simulink model "hip_controller_2026_01_07"  (R2024b)
settings: Solver=FixedStepAuto  StartTime=0.0  StopTime=simDuration  FixedStep=0.01  RelTol=1e-3  EnableMultiTasking=on
InitFcn:
  | breakp=[-1, -0.8, -0.6, -0.4, -0.2, -0.1, 0, 0.1, 0.2, 0.4, 0.6, 0.8, 1];
  | splinenew =[-1, -0.8, -0.6, -0.4, -0.2, -0.1, 0, 0, 0.005, 0.01, 0.015,0.02,0.025];
undefined symbols (not defined in the file or in its folder): Discrete, K, qbreak, Time
libraries: simulink x53, arduinolib x11, dspswit3 x9, ctrlSharedLib x4, dspfdesign x2, slpidlib x2
(part 3 of 4)

== system hip_controller_2026_01_07/Subsystem3/Left Motor Velocity/Motor Actual Position Receive/CHINESE CORRECTION ==
  position : Inport
  Enable : EnablePort  StatesWhenEnabling=reset
  Abs : Abs  SaturateOnIntegerOverflow=off
  Constant2 : Constant
  Constant3 : Constant  Value=0
  Memory : Memory
  Subsystem : Subsystem
  Sum : Sum  Inputs=|+-
  Sum1 : Sum  Inputs=+-
  Switch1 : Switch  Criteria=u2 > Threshold  Threshold=20  SaturateOnIntegerOverflow=off  InputSameDT=off
  Out1 : Outport
  wires:
  Constant2/1 -> Switch1/1
  position/1 -> Sum1/1, Sum/1, Memory/1
  Sum/1 -> Abs/1, Subsystem/1(In1)
  Sum1/1 -> Out1/1
  Abs/1 -> Switch1/2
  Constant3/1 -> Switch1/3
  Switch1/1 -> Subsystem/Enable
  Memory/1 -> Sum/2
  Subsystem/1(Out1) -> Sum1/2

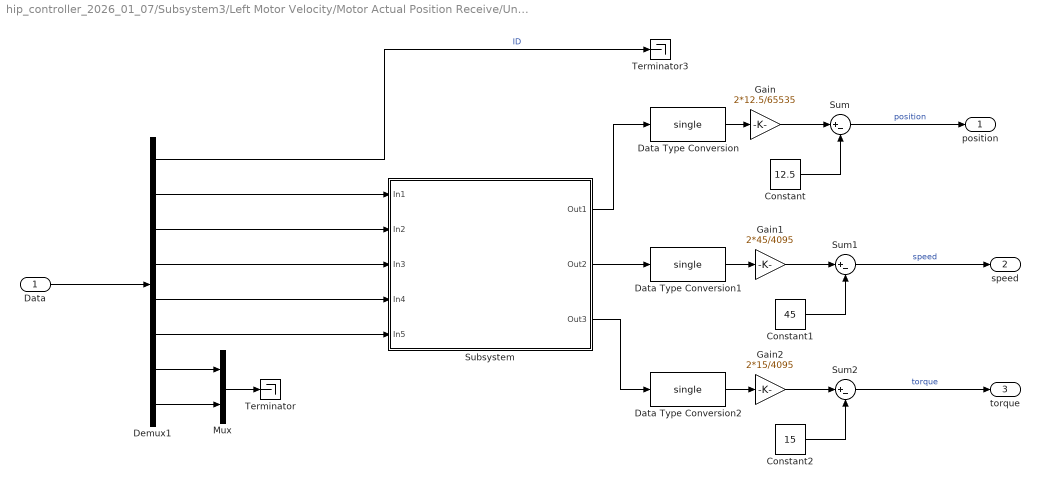
== system hip_controller_2026_01_07/Subsystem3/Left Motor Velocity/Motor Actual Position Receive/Unpack2 ==
  Data : Inport
  Constant : Constant  Value=12.5
  Constant1 : Constant  Value=45
  Constant2 : Constant  Value=15
  Data Type Conversion : DataTypeConversion  OutDataTypeStr=single  SaturateOnIntegerOverflow=off  RndMeth=Floor
  Data Type Conversion1 : DataTypeConversion  OutDataTypeStr=single  SaturateOnIntegerOverflow=off  RndMeth=Floor
  Data Type Conversion2 : DataTypeConversion  OutDataTypeStr=single  SaturateOnIntegerOverflow=off  RndMeth=Floor
  Demux1 : Demux  Outputs=8
  Gain : Gain  Gain=2*12.5/65535  RndMeth=Round
  Gain1 : Gain  Gain=2*45/4095  RndMeth=Round
  Gain2 : Gain  Gain=2*15/4095  RndMeth=Round
  Mux : Mux  Inputs=2
  Subsystem : Subsystem
  Sum : Sum  Inputs=|+-
  Sum1 : Sum  Inputs=|+-
  Sum2 : Sum  Inputs=|+-
  Terminator : Terminator
  Terminator3 : Terminator
  position : Outport
  speed : Outport  Port=2
  torque : Outport  Port=3
  wires:
  Demux1/1 -> Terminator3/1  "ID"
  Demux1/7 -> Mux/1
  Demux1/8 -> Mux/2
  Demux1/2 -> Subsystem/1(In1)
  Demux1/3 -> Subsystem/2(In2)
  Demux1/4 -> Subsystem/3(In3)
  Demux1/5 -> Subsystem/4(In4)
  Demux1/6 -> Subsystem/5(In5)
  Subsystem/1(Out1) -> Data Type Conversion/1
  Gain/1 -> Sum/1
  Constant/1 -> Sum/2
  Data Type Conversion/1 -> Gain/1
  Gain1/1 -> Sum1/1
  Data Type Conversion1/1 -> Gain1/1
  Constant1/1 -> Sum1/2
  Gain2/1 -> Sum2/1
  Data Type Conversion2/1 -> Gain2/1
  Constant2/1 -> Sum2/2
  Subsystem/2(Out2) -> Data Type Conversion1/1
  Subsystem/3(Out3) -> Data Type Conversion2/1
  Sum2/1 -> torque/1  "torque"
  Mux/1 -> Terminator/1
  Data/1 -> Demux1/1
  Sum/1 -> position/1  "position"
  Sum1/1 -> speed/1  "speed"

== system hip_controller_2026_01_07/Subsystem3/Left Motor Velocity/Subsystem/CAN Pack1 ==
  Position : Inport
  Velocity : Inport  Port=2
  Kp : Inport  Port=3
  Kd : Inport  Port=4
  Torque : Inport  Port=5
  Constant3 : Constant  Value=-12.5  OutDataTypeStr=single
  Constant4 : Constant  Value=-45  OutDataTypeStr=single
  Constant5 : Constant  Value=-15  OutDataTypeStr=single
  Gain : Gain  Gain=65535/(2*12.5)  OutDataTypeStr=uint16  RndMeth=Round
  Gain3 : Gain  Gain=4095/(2*45)  OutDataTypeStr=fixdt(0,12,0)  RndMeth=Round
  Gain4 : Gain  Gain=4095/500  OutDataTypeStr=fixdt(0,12,0)  RndMeth=Round
  Gain5 : Gain  Gain=4095/5  OutDataTypeStr=fixdt(0,12,0)  RndMeth=Round
  Gain6 : Gain  Gain=4095/(2*15)  OutDataTypeStr=fixdt(0,12,0)  RndMeth=Round
  Subsystem : Subsystem
  Sum3 : Sum  Inputs=|+-
  Sum4 : Sum  Inputs=|+-
  Sum5 : Sum  Inputs=|+-
  Vector Concatenate : Concatenate  NumInputs=8
  CAN Data : Outport
  wires:
  Velocity/1 -> Sum4/1
  Kp/1 -> Gain4/1
  Kd/1 -> Gain5/1
  Vector Concatenate/1 -> CAN Data/1
  Constant3/1 -> Sum3/2
  Sum3/1 -> Gain/1  "position"
  Position/1 -> Sum3/1
  Constant4/1 -> Sum4/2
  Constant5/1 -> Sum5/2
  Sum5/1 -> Gain6/1  "torque"
  Torque/1 -> Sum5/1
  Sum4/1 -> Gain3/1  "speed"
  Gain/1 -> Subsystem/1(p_int)
  Gain3/1 -> Subsystem/2(v_int)
  Gain4/1 -> Subsystem/3(kp_int)
  Gain5/1 -> Subsystem/4(kd_int)
  Gain6/1 -> Subsystem/5(t_int)
  Subsystem/1(Out2) -> Vector Concatenate/1
  Subsystem/2(Out1) -> Vector Concatenate/2
  Subsystem/4(Out4) -> Vector Concatenate/4
  Subsystem/5(Out5) -> Vector Concatenate/5
  Subsystem/6(Out6) -> Vector Concatenate/6
  Subsystem/7(Out7) -> Vector Concatenate/7
  Subsystem/3(Out3) -> Vector Concatenate/3
  Subsystem/8(Out8) -> Vector Concatenate/8

== system hip_controller_2026_01_07/Subsystem3/Left Motor Velocity/Subsystem/Subsystem2 ==
  Enable : Inport
  Velocity : Inport  Port=2
  Mux1 : Mux  Inputs=5
  Subsystem : Subsystem
  Subsystem2 : Subsystem
  Enter_motor_mode : Outport
  Velocity_value : Outport  Port=2
  wires:
  Subsystem2/3(Out3) -> Mux1/3
  Subsystem2/2(Out2) -> Mux1/2
  Subsystem2/4(Out4) -> Mux1/4
  Subsystem2/1(Out1) -> Mux1/1
  Subsystem/1(Out1) -> Velocity_value/1
  Mux1/1 -> Enter_motor_mode/1
  Enable/1 -> Mux1/5
  Velocity/1 -> Subsystem/1(In1)

== system hip_controller_2026_01_07/Subsystem3/Right Motor Velocity/Motor Actual Position Receive/CHINESE CORRECTION ==
  position : Inport
  Enable : EnablePort  StatesWhenEnabling=reset
  Abs : Abs  SaturateOnIntegerOverflow=off
  Constant2 : Constant
  Constant3 : Constant  Value=0
  Memory : Memory
  Subsystem : Subsystem
  Sum : Sum  Inputs=|+-
  Sum1 : Sum  Inputs=+-
  Switch1 : Switch  Criteria=u2 > Threshold  Threshold=20  SaturateOnIntegerOverflow=off  InputSameDT=off
  Out1 : Outport
  wires:
  Constant2/1 -> Switch1/1
  position/1 -> Sum1/1, Sum/1, Memory/1
  Sum/1 -> Abs/1, Subsystem/1(In1)
  Sum1/1 -> Out1/1
  Abs/1 -> Switch1/2
  Constant3/1 -> Switch1/3
  Switch1/1 -> Subsystem/Enable
  Memory/1 -> Sum/2
  Subsystem/1(Out1) -> Sum1/2

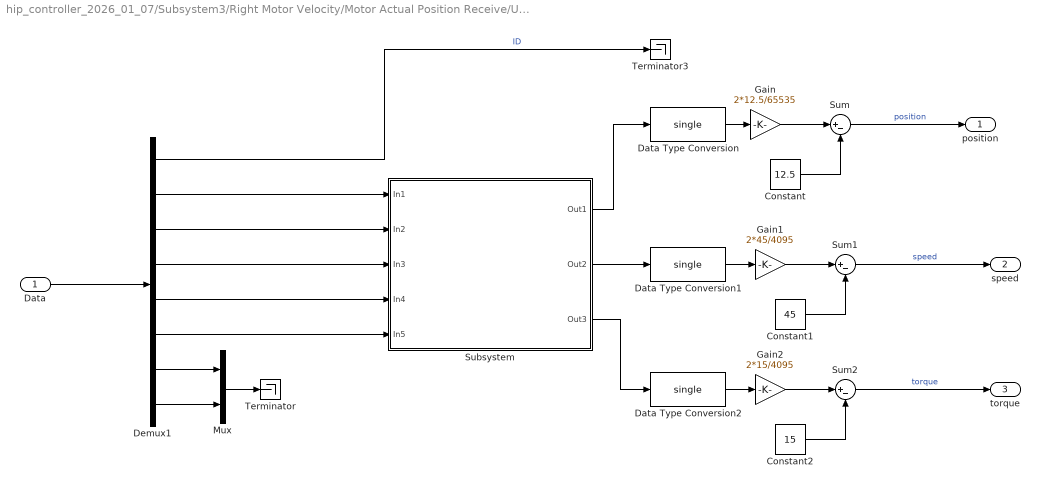
== system hip_controller_2026_01_07/Subsystem3/Right Motor Velocity/Motor Actual Position Receive/Unpack2 ==
  Data : Inport
  Constant : Constant  Value=12.5
  Constant1 : Constant  Value=45
  Constant2 : Constant  Value=15
  Data Type Conversion : DataTypeConversion  OutDataTypeStr=single  SaturateOnIntegerOverflow=off  RndMeth=Floor
  Data Type Conversion1 : DataTypeConversion  OutDataTypeStr=single  SaturateOnIntegerOverflow=off  RndMeth=Floor
  Data Type Conversion2 : DataTypeConversion  OutDataTypeStr=single  SaturateOnIntegerOverflow=off  RndMeth=Floor
  Demux1 : Demux  Outputs=8
  Gain : Gain  Gain=2*12.5/65535  RndMeth=Round
  Gain1 : Gain  Gain=2*45/4095  RndMeth=Round
  Gain2 : Gain  Gain=2*15/4095  RndMeth=Round
  Mux : Mux  Inputs=2
  Subsystem : Subsystem
  Sum : Sum  Inputs=|+-
  Sum1 : Sum  Inputs=|+-
  Sum2 : Sum  Inputs=|+-
  Terminator : Terminator
  Terminator3 : Terminator
  position : Outport
  speed : Outport  Port=2
  torque : Outport  Port=3
  wires:
  Demux1/1 -> Terminator3/1  "ID"
  Demux1/7 -> Mux/1
  Demux1/8 -> Mux/2
  Demux1/2 -> Subsystem/1(In1)
  Demux1/3 -> Subsystem/2(In2)
  Demux1/4 -> Subsystem/3(In3)
  Demux1/5 -> Subsystem/4(In4)
  Demux1/6 -> Subsystem/5(In5)
  Subsystem/1(Out1) -> Data Type Conversion/1
  Gain/1 -> Sum/1
  Constant/1 -> Sum/2
  Data Type Conversion/1 -> Gain/1
  Gain1/1 -> Sum1/1
  Data Type Conversion1/1 -> Gain1/1
  Constant1/1 -> Sum1/2
  Gain2/1 -> Sum2/1
  Data Type Conversion2/1 -> Gain2/1
  Constant2/1 -> Sum2/2
  Subsystem/2(Out2) -> Data Type Conversion1/1
  Subsystem/3(Out3) -> Data Type Conversion2/1
  Sum2/1 -> torque/1  "torque"
  Mux/1 -> Terminator/1
  Data/1 -> Demux1/1
  Sum/1 -> position/1  "position"
  Sum1/1 -> speed/1  "speed"

== system hip_controller_2026_01_07/Subsystem3/Right Motor Velocity/Subsystem/CAN Pack1 ==
  Position : Inport
  Velocity : Inport  Port=2
  Kp : Inport  Port=3
  Kd : Inport  Port=4
  Torque : Inport  Port=5
  Constant3 : Constant  Value=-12.5  OutDataTypeStr=single
  Constant4 : Constant  Value=-45  OutDataTypeStr=single
  Constant5 : Constant  Value=-15  OutDataTypeStr=single
  Gain : Gain  Gain=65535/(2*12.5)  OutDataTypeStr=uint16  RndMeth=Round
  Gain3 : Gain  Gain=4095/(2*45)  OutDataTypeStr=fixdt(0,12,0)  RndMeth=Round
  Gain4 : Gain  Gain=4095/500  OutDataTypeStr=fixdt(0,12,0)  RndMeth=Round
  Gain5 : Gain  Gain=4095/5  OutDataTypeStr=fixdt(0,12,0)  RndMeth=Round
  Gain6 : Gain  Gain=4095/(2*15)  OutDataTypeStr=fixdt(0,12,0)  RndMeth=Round
  Subsystem : Subsystem
  Sum3 : Sum  Inputs=|+-
  Sum4 : Sum  Inputs=|+-
  Sum5 : Sum  Inputs=|+-
  Vector Concatenate : Concatenate  NumInputs=8
  CAN Data : Outport
  wires:
  Velocity/1 -> Sum4/1
  Kp/1 -> Gain4/1
  Kd/1 -> Gain5/1
  Vector Concatenate/1 -> CAN Data/1
  Constant3/1 -> Sum3/2
  Sum3/1 -> Gain/1  "position"
  Position/1 -> Sum3/1
  Constant4/1 -> Sum4/2
  Constant5/1 -> Sum5/2
  Sum5/1 -> Gain6/1  "torque"
  Torque/1 -> Sum5/1
  Sum4/1 -> Gain3/1  "speed"
  Gain/1 -> Subsystem/1(p_int)
  Gain3/1 -> Subsystem/2(v_int)
  Gain4/1 -> Subsystem/3(kp_int)
  Gain5/1 -> Subsystem/4(kd_int)
  Gain6/1 -> Subsystem/5(t_int)
  Subsystem/1(Out2) -> Vector Concatenate/1
  Subsystem/2(Out1) -> Vector Concatenate/2
  Subsystem/4(Out4) -> Vector Concatenate/4
  Subsystem/5(Out5) -> Vector Concatenate/5
  Subsystem/6(Out6) -> Vector Concatenate/6
  Subsystem/7(Out7) -> Vector Concatenate/7
  Subsystem/3(Out3) -> Vector Concatenate/3
  Subsystem/8(Out8) -> Vector Concatenate/8

== system hip_controller_2026_01_07/Subsystem3/Right Motor Velocity/Subsystem/Subsystem2 ==
  Enable : Inport
  Velocity : Inport  Port=2
  Mux1 : Mux  Inputs=5
  Subsystem : Subsystem
  Subsystem2 : Subsystem
  Enter_motor_mode : Outport
  Velocity_value : Outport  Port=2
  wires:
  Subsystem2/3(Out3) -> Mux1/3
  Subsystem2/2(Out2) -> Mux1/2
  Subsystem2/4(Out4) -> Mux1/4
  Subsystem2/1(Out1) -> Mux1/1
  Subsystem/1(Out1) -> Velocity_value/1
  Mux1/1 -> Enter_motor_mode/1
  Enable/1 -> Mux1/5
  Velocity/1 -> Subsystem/1(In1)

== system hip_controller_2026_01_07/Subsystem4/Left Motor Velocity/Motor Actual Position Receive/CHINESE CORRECTION ==
  position : Inport
  Enable : EnablePort  StatesWhenEnabling=reset
  Abs : Abs  SaturateOnIntegerOverflow=off
  Constant2 : Constant
  Constant3 : Constant  Value=0
  Memory : Memory
  Subsystem : Subsystem
  Sum : Sum  Inputs=|+-
  Sum1 : Sum  Inputs=+-
  Switch1 : Switch  Criteria=u2 > Threshold  Threshold=20  SaturateOnIntegerOverflow=off  InputSameDT=off
  Out1 : Outport
  wires:
  Constant2/1 -> Switch1/1
  position/1 -> Sum1/1, Sum/1, Memory/1
  Sum/1 -> Abs/1, Subsystem/1(In1)
  Sum1/1 -> Out1/1
  Abs/1 -> Switch1/2
  Constant3/1 -> Switch1/3
  Switch1/1 -> Subsystem/Enable
  Memory/1 -> Sum/2
  Subsystem/1(Out1) -> Sum1/2

== system hip_controller_2026_01_07/Subsystem4/Left Motor Velocity/Motor Actual Position Receive/Unpack2 ==
  Data : Inport
  Constant : Constant  Value=12.5
  Constant1 : Constant  Value=45
  Constant2 : Constant  Value=15
  Data Type Conversion : DataTypeConversion  OutDataTypeStr=single  SaturateOnIntegerOverflow=off  RndMeth=Floor
  Data Type Conversion1 : DataTypeConversion  OutDataTypeStr=single  SaturateOnIntegerOverflow=off  RndMeth=Floor
  Data Type Conversion2 : DataTypeConversion  OutDataTypeStr=single  SaturateOnIntegerOverflow=off  RndMeth=Floor
  Demux1 : Demux  Outputs=8
  Gain : Gain  Gain=2*12.5/65535  RndMeth=Round
  Gain1 : Gain  Gain=2*45/4095  RndMeth=Round
  Gain2 : Gain  Gain=2*15/4095  RndMeth=Round
  Mux : Mux  Inputs=2
  Subsystem : Subsystem
  Sum : Sum  Inputs=|+-
  Sum1 : Sum  Inputs=|+-
  Sum2 : Sum  Inputs=|+-
  Terminator : Terminator
  Terminator3 : Terminator
  position : Outport
  speed : Outport  Port=2
  torque : Outport  Port=3
  wires:
  Demux1/1 -> Terminator3/1  "ID"
  Demux1/7 -> Mux/1
  Demux1/8 -> Mux/2
  Demux1/2 -> Subsystem/1(In1)
  Demux1/3 -> Subsystem/2(In2)
  Demux1/4 -> Subsystem/3(In3)
  Demux1/5 -> Subsystem/4(In4)
  Demux1/6 -> Subsystem/5(In5)
  Subsystem/1(Out1) -> Data Type Conversion/1
  Gain/1 -> Sum/1
  Constant/1 -> Sum/2
  Data Type Conversion/1 -> Gain/1
  Gain1/1 -> Sum1/1
  Data Type Conversion1/1 -> Gain1/1
  Constant1/1 -> Sum1/2
  Gain2/1 -> Sum2/1
  Data Type Conversion2/1 -> Gain2/1
  Constant2/1 -> Sum2/2
  Subsystem/2(Out2) -> Data Type Conversion1/1
  Subsystem/3(Out3) -> Data Type Conversion2/1
  Sum2/1 -> torque/1  "torque"
  Mux/1 -> Terminator/1
  Data/1 -> Demux1/1
  Sum/1 -> position/1  "position"
  Sum1/1 -> speed/1  "speed"

== system hip_controller_2026_01_07/Subsystem4/Left Motor Velocity/Subsystem/CAN Pack1 ==
  Position : Inport
  Velocity : Inport  Port=2
  Kp : Inport  Port=3
  Kd : Inport  Port=4
  Torque : Inport  Port=5
  Constant3 : Constant  Value=-12.5  OutDataTypeStr=single
  Constant4 : Constant  Value=-45  OutDataTypeStr=single
  Constant5 : Constant  Value=-15  OutDataTypeStr=single
  Gain : Gain  Gain=65535/(2*12.5)  OutDataTypeStr=uint16  RndMeth=Round
  Gain3 : Gain  Gain=4095/(2*45)  OutDataTypeStr=fixdt(0,12,0)  RndMeth=Round
  Gain4 : Gain  Gain=4095/500  OutDataTypeStr=fixdt(0,12,0)  RndMeth=Round
  Gain5 : Gain  Gain=4095/5  OutDataTypeStr=fixdt(0,12,0)  RndMeth=Round
  Gain6 : Gain  Gain=4095/(2*15)  OutDataTypeStr=fixdt(0,12,0)  RndMeth=Round
  Subsystem : Subsystem
  Sum3 : Sum  Inputs=|+-
  Sum4 : Sum  Inputs=|+-
  Sum5 : Sum  Inputs=|+-
  Vector Concatenate : Concatenate  NumInputs=8
  CAN Data : Outport
  wires:
  Velocity/1 -> Sum4/1
  Kp/1 -> Gain4/1
  Kd/1 -> Gain5/1
  Vector Concatenate/1 -> CAN Data/1
  Constant3/1 -> Sum3/2
  Sum3/1 -> Gain/1  "position"
  Position/1 -> Sum3/1
  Constant4/1 -> Sum4/2
  Constant5/1 -> Sum5/2
  Sum5/1 -> Gain6/1  "torque"
  Torque/1 -> Sum5/1
  Sum4/1 -> Gain3/1  "speed"
  Gain/1 -> Subsystem/1(p_int)
  Gain3/1 -> Subsystem/2(v_int)
  Gain4/1 -> Subsystem/3(kp_int)
  Gain5/1 -> Subsystem/4(kd_int)
  Gain6/1 -> Subsystem/5(t_int)
  Subsystem/1(Out2) -> Vector Concatenate/1
  Subsystem/2(Out1) -> Vector Concatenate/2
  Subsystem/4(Out4) -> Vector Concatenate/4
  Subsystem/5(Out5) -> Vector Concatenate/5
  Subsystem/6(Out6) -> Vector Concatenate/6
  Subsystem/7(Out7) -> Vector Concatenate/7
  Subsystem/3(Out3) -> Vector Concatenate/3
  Subsystem/8(Out8) -> Vector Concatenate/8

== system hip_controller_2026_01_07/Subsystem4/Left Motor Velocity/Subsystem/Subsystem2 ==
  Enable : Inport
  Velocity : Inport  Port=2
  Mux1 : Mux  Inputs=5
  Subsystem : Subsystem
  Subsystem2 : Subsystem
  Enter_motor_mode : Outport
  Velocity_value : Outport  Port=2
  wires:
  Subsystem2/3(Out3) -> Mux1/3
  Subsystem2/2(Out2) -> Mux1/2
  Subsystem2/4(Out4) -> Mux1/4
  Subsystem2/1(Out1) -> Mux1/1
  Subsystem/1(Out1) -> Velocity_value/1
  Mux1/1 -> Enter_motor_mode/1
  Enable/1 -> Mux1/5
  Velocity/1 -> Subsystem/1(In1)

== system hip_controller_2026_01_07/Subsystem4/Right Motor Velocity/Motor Actual Position Receive/CHINESE CORRECTION ==
  position : Inport
  Enable : EnablePort  StatesWhenEnabling=reset
  Abs : Abs  SaturateOnIntegerOverflow=off
  Constant2 : Constant
  Constant3 : Constant  Value=0
  Memory : Memory
  Subsystem : Subsystem
  Sum : Sum  Inputs=|+-
  Sum1 : Sum  Inputs=+-
  Switch1 : Switch  Criteria=u2 > Threshold  Threshold=20  SaturateOnIntegerOverflow=off  InputSameDT=off
  Out1 : Outport
  wires:
  Constant2/1 -> Switch1/1
  position/1 -> Sum1/1, Sum/1, Memory/1
  Sum/1 -> Abs/1, Subsystem/1(In1)
  Sum1/1 -> Out1/1
  Abs/1 -> Switch1/2
  Constant3/1 -> Switch1/3
  Switch1/1 -> Subsystem/Enable
  Memory/1 -> Sum/2
  Subsystem/1(Out1) -> Sum1/2

== system hip_controller_2026_01_07/Subsystem4/Right Motor Velocity/Motor Actual Position Receive/Unpack2 ==
  Data : Inport
  Constant : Constant  Value=12.5
  Constant1 : Constant  Value=45
  Constant2 : Constant  Value=15
  Data Type Conversion : DataTypeConversion  OutDataTypeStr=single  SaturateOnIntegerOverflow=off  RndMeth=Floor
  Data Type Conversion1 : DataTypeConversion  OutDataTypeStr=single  SaturateOnIntegerOverflow=off  RndMeth=Floor
  Data Type Conversion2 : DataTypeConversion  OutDataTypeStr=single  SaturateOnIntegerOverflow=off  RndMeth=Floor
  Demux1 : Demux  Outputs=8
  Gain : Gain  Gain=2*12.5/65535  RndMeth=Round
  Gain1 : Gain  Gain=2*45/4095  RndMeth=Round
  Gain2 : Gain  Gain=2*15/4095  RndMeth=Round
  Mux : Mux  Inputs=2
  Subsystem : Subsystem
  Sum : Sum  Inputs=|+-
  Sum1 : Sum  Inputs=|+-
  Sum2 : Sum  Inputs=|+-
  Terminator : Terminator
  Terminator3 : Terminator
  position : Outport
  speed : Outport  Port=2
  torque : Outport  Port=3
  wires:
  Demux1/1 -> Terminator3/1  "ID"
  Demux1/7 -> Mux/1
  Demux1/8 -> Mux/2
  Demux1/2 -> Subsystem/1(In1)
  Demux1/3 -> Subsystem/2(In2)
  Demux1/4 -> Subsystem/3(In3)
  Demux1/5 -> Subsystem/4(In4)
  Demux1/6 -> Subsystem/5(In5)
  Subsystem/1(Out1) -> Data Type Conversion/1
  Gain/1 -> Sum/1
  Constant/1 -> Sum/2
  Data Type Conversion/1 -> Gain/1
  Gain1/1 -> Sum1/1
  Data Type Conversion1/1 -> Gain1/1
  Constant1/1 -> Sum1/2
  Gain2/1 -> Sum2/1
  Data Type Conversion2/1 -> Gain2/1
  Constant2/1 -> Sum2/2
  Subsystem/2(Out2) -> Data Type Conversion1/1
  Subsystem/3(Out3) -> Data Type Conversion2/1
  Sum2/1 -> torque/1  "torque"
  Mux/1 -> Terminator/1
  Data/1 -> Demux1/1
  Sum/1 -> position/1  "position"
  Sum1/1 -> speed/1  "speed"

== system hip_controller_2026_01_07/Subsystem4/Right Motor Velocity/Subsystem/CAN Pack1 ==
  Position : Inport
  Velocity : Inport  Port=2
  Kp : Inport  Port=3
  Kd : Inport  Port=4
  Torque : Inport  Port=5
  Constant3 : Constant  Value=-12.5  OutDataTypeStr=single
  Constant4 : Constant  Value=-45  OutDataTypeStr=single
  Constant5 : Constant  Value=-15  OutDataTypeStr=single
  Gain : Gain  Gain=65535/(2*12.5)  OutDataTypeStr=uint16  RndMeth=Round
  Gain3 : Gain  Gain=4095/(2*45)  OutDataTypeStr=fixdt(0,12,0)  RndMeth=Round
  Gain4 : Gain  Gain=4095/500  OutDataTypeStr=fixdt(0,12,0)  RndMeth=Round
  Gain5 : Gain  Gain=4095/5  OutDataTypeStr=fixdt(0,12,0)  RndMeth=Round
  Gain6 : Gain  Gain=4095/(2*15)  OutDataTypeStr=fixdt(0,12,0)  RndMeth=Round
  Subsystem : Subsystem
  Sum3 : Sum  Inputs=|+-
  Sum4 : Sum  Inputs=|+-
  Sum5 : Sum  Inputs=|+-
  Vector Concatenate : Concatenate  NumInputs=8
  CAN Data : Outport
  wires:
  Velocity/1 -> Sum4/1
  Kp/1 -> Gain4/1
  Kd/1 -> Gain5/1
  Vector Concatenate/1 -> CAN Data/1
  Constant3/1 -> Sum3/2
  Sum3/1 -> Gain/1  "position"
  Position/1 -> Sum3/1
  Constant4/1 -> Sum4/2
  Constant5/1 -> Sum5/2
  Sum5/1 -> Gain6/1  "torque"
  Torque/1 -> Sum5/1
  Sum4/1 -> Gain3/1  "speed"
  Gain/1 -> Subsystem/1(p_int)
  Gain3/1 -> Subsystem/2(v_int)
  Gain4/1 -> Subsystem/3(kp_int)
  Gain5/1 -> Subsystem/4(kd_int)
  Gain6/1 -> Subsystem/5(t_int)
  Subsystem/1(Out2) -> Vector Concatenate/1
  Subsystem/2(Out1) -> Vector Concatenate/2
  Subsystem/4(Out4) -> Vector Concatenate/4
  Subsystem/5(Out5) -> Vector Concatenate/5
  Subsystem/6(Out6) -> Vector Concatenate/6
  Subsystem/7(Out7) -> Vector Concatenate/7
  Subsystem/3(Out3) -> Vector Concatenate/3
  Subsystem/8(Out8) -> Vector Concatenate/8

== system hip_controller_2026_01_07/Subsystem4/Right Motor Velocity/Subsystem/Subsystem2 ==
  Enable : Inport
  Velocity : Inport  Port=2
  Mux1 : Mux  Inputs=5
  Subsystem : Subsystem
  Subsystem2 : Subsystem
  Enter_motor_mode : Outport
  Velocity_value : Outport  Port=2
  wires:
  Subsystem2/3(Out3) -> Mux1/3
  Subsystem2/2(Out2) -> Mux1/2
  Subsystem2/4(Out4) -> Mux1/4
  Subsystem2/1(Out1) -> Mux1/1
  Subsystem/1(Out1) -> Velocity_value/1
  Mux1/1 -> Enter_motor_mode/1
  Enable/1 -> Mux1/5
  Velocity/1 -> Subsystem/1(In1)

== system hip_controller_2026_01_07/LEFT LEG1/Pos and Vel normalized/Subsystem4/If Action Subsystem/Enabled Subsystem ==
  angle_in : Inport
  Enable : EnablePort
  angle_out : Outport
  wires:
  angle_in/1 -> angle_out/1

== system hip_controller_2026_01_07/LEFT LEG1/Pos and Vel normalized/Subsystem5/If Action Subsystem/Enabled Subsystem ==
  angle_in : Inport
  Enable : EnablePort
  angle_out : Outport
  wires:
  angle_in/1 -> angle_out/1

== system hip_controller_2026_01_07/LEFT LEG1/Pos and Vel normalized/Subsystem6/If Action Subsystem/Enabled Subsystem ==
  vel_in : Inport
  Enable : EnablePort
  vel_out : Outport
  wires:
  vel_in/1 -> vel_out/1

== system hip_controller_2026_01_07/LEFT LEG1/Pos and Vel normalized/Subsystem7/If Action Subsystem/Enabled Subsystem ==
  vel_in : Inport
  Enable : EnablePort
  vel_out : Outport
  wires:
  vel_in/1 -> vel_out/1

== system hip_controller_2026_01_07/RIGHT_LEG1/Pos and Vel normalized/Subsystem4/If Action Subsystem/Enabled Subsystem ==
  angle_in : Inport
  Enable : EnablePort
  angle_out : Outport
  wires:
  angle_in/1 -> angle_out/1

== system hip_controller_2026_01_07/RIGHT_LEG1/Pos and Vel normalized/Subsystem5/If Action Subsystem/Enabled Subsystem ==
  angle_in : Inport
  Enable : EnablePort
  angle_out : Outport
  wires:
  angle_in/1 -> angle_out/1

== system hip_controller_2026_01_07/RIGHT_LEG1/Pos and Vel normalized/Subsystem6/If Action Subsystem/Enabled Subsystem ==
  vel_in : Inport
  Enable : EnablePort
  vel_out : Outport
  wires:
  vel_in/1 -> vel_out/1

== system hip_controller_2026_01_07/RIGHT_LEG1/Pos and Vel normalized/Subsystem7/If Action Subsystem/Enabled Subsystem ==
  vel_in : Inport
  Enable : EnablePort
  vel_out : Outport
  wires:
  vel_in/1 -> vel_out/1

== system hip_controller_2026_01_07/Subsystem3/Left Motor Velocity/Motor Actual Position Receive/CHINESE CORRECTION/Subsystem ==
  In1 : Inport
  Enable : EnablePort
  Memory : Memory
  Sum : Sum  Inputs=|++
  Out1 : Outport
  wires:
  In1/1 -> Sum/1
  Sum/1 -> Out1/1, Memory/1
  Memory/1 -> Sum/2

== system hip_controller_2026_01_07/Subsystem3/Left Motor Velocity/Motor Actual Position Receive/Unpack2/Subsystem ==
  In1 : Inport
  In2 : Inport  Port=2
  In3 : Inport  Port=3
  In4 : Inport  Port=4
  In5 : Inport  Port=5
  Bitwise AND : simulink/Logic and Bit Operations/Bitwise Operator  logicop=AND  UseBitMask=on  BitMask=bin2dec('0000000000001111')  BitMaskRealWorld=Stored Integer
  Bitwise OR : simulink/Logic and Bit Operations/Bitwise Operator  logicop=OR  UseBitMask=off  NumInputPorts=2  BitMask=bin2dec('11011001')  BitMaskRealWorld=Stored Integer
  Bitwise OR1 : simulink/Logic and Bit Operations/Bitwise Operator  logicop=OR  UseBitMask=off  NumInputPorts=2  BitMask=bin2dec('11011001')  BitMaskRealWorld=Stored Integer
  Bitwise OR2 : simulink/Logic and Bit Operations/Bitwise Operator  logicop=OR  UseBitMask=off  NumInputPorts=2  BitMask=bin2dec('11011001')  BitMaskRealWorld=Stored Integer
  Constant : Constant  Value=8  OutDataTypeStr=uint16
  Constant1 : Constant  Value=4  OutDataTypeStr=uint16
  Constant2 : Constant  Value=4  OutDataTypeStr=uint16
  Constant4 : Constant  Value=8  OutDataTypeStr=uint16
  Shift Arithmetic1 : ArithShift  BitShiftNumberSource=Input port  BitShiftNumber=8  BitShiftDirection=Left
      settings: InputPortMap=u0,p1
  Shift Arithmetic2 : ArithShift  BitShiftNumberSource=Input port  BitShiftNumber=8  BitShiftDirection=Left
      settings: InputPortMap=u0,p1
  Shift Arithmetic3 : ArithShift  BitShiftNumberSource=Input port  BitShiftNumber=8  BitShiftDirection=Right
      settings: InputPortMap=u0,p1
  Shift Arithmetic4 : ArithShift  BitShiftNumberSource=Input port  BitShiftNumber=8  BitShiftDirection=Left
      settings: InputPortMap=u0,p1
  Out1 : Outport
  Out2 : Outport  Port=2
  Out3 : Outport  Port=3
  wires:
  Bitwise AND/1 -> Shift Arithmetic4/1
  In5/1 -> Bitwise OR2/1
  Shift Arithmetic1/1 -> Bitwise OR1/1
  In1/1 -> Shift Arithmetic1/1
  Shift Arithmetic2/1 -> Bitwise OR/1
  Shift Arithmetic3/1 -> Bitwise OR/2
  Shift Arithmetic4/1 -> Bitwise OR2/2
  In2/1 -> Bitwise OR1/2
  Bitwise OR1/1 -> Out1/1
  Bitwise OR2/1 -> Out3/1
  In3/1 -> Shift Arithmetic2/1
  Constant4/1 -> Shift Arithmetic4/2
  Constant2/1 -> Shift Arithmetic3/2
  Constant1/1 -> Shift Arithmetic2/2
  Constant/1 -> Shift Arithmetic1/2
  Bitwise OR/1 -> Out2/1
  In4/1 -> Shift Arithmetic3/1, Bitwise AND/1

== system hip_controller_2026_01_07/Subsystem3/Left Motor Velocity/Subsystem/CAN Pack1/Subsystem ==
  p_int : Inport
  v_int : Inport  Port=2
  kp_int : Inport  Port=3
  kd_int : Inport  Port=4
  t_int : Inport  Port=5
  Buff 0 : Subsystem
  Buff 1 : Subsystem
  Buff 2 : Subsystem
  Buff 3 : Subsystem
  Buff 4 : Subsystem
  Buff 5 : Subsystem
  Buff 6 : Subsystem
  Buff 7 : Subsystem
  Out2 : Outport
  Out1 : Outport  Port=2
  Out3 : Outport  Port=3
  Out4 : Outport  Port=4
  Out5 : Outport  Port=5
  Out6 : Outport  Port=6
  Out7 : Outport  Port=7
  Out8 : Outport  Port=8
  wires:
  Buff 5/1(Out1) -> Out6/1
  Buff 7/1(Out1) -> Out8/1
  Buff 6/1(Out1) -> Out7/1
  Buff 0/1(Out1) -> Out2/1
  Buff 1/1(Out1) -> Out1/1
  Buff 2/1(Out1) -> Out3/1
  Buff 4/1(Out1) -> Out5/1
  Buff 3/1(Out1) -> Out4/1
  p_int/1 -> Buff 0/1(In1), Buff 1/1(In1)
  v_int/1 -> Buff 3/1(In1), Buff 2/1(In1)
  kd_int/1 -> Buff 6/1(In3), Buff 5/1(In2)
  kp_int/1 -> Buff 3/2(In2), Buff 4/1(In1)
  t_int/1 -> Buff 7/1(In1), Buff 6/2(In4)

== system hip_controller_2026_01_07/Subsystem3/Left Motor Velocity/Subsystem/Subsystem2/Subsystem ==
  In1 : Inport
  Kd : Constant  OutDataTypeStr=single
  Kp : Constant  Value=0  OutDataTypeStr=single
  Mux2 : Mux  Inputs=5
  Position Command : Constant  Value=0  VectorParams1D=off  OutDataTypeStr=single
  Saturation : Saturate  UpperLimit=12.5  LowerLimit=-12.5
  Saturation1 : Saturate  UpperLimit=41.87  LowerLimit=-41.87
  Saturation2 : Saturate  UpperLimit=500  LowerLimit=0
  Saturation3 : Saturate  UpperLimit=5  LowerLimit=0
  Saturation4 : Saturate  UpperLimit=9  LowerLimit=-9
  Torque : Constant  Value=0  OutDataTypeStr=single
  Out1 : Outport
  wires:
  Saturation/1 -> Mux2/1
  Kp/1 -> Saturation2/1
  In1/1 -> Saturation1/1
  Position Command/1 -> Saturation/1
  Saturation1/1 -> Mux2/2
  Kd/1 -> Saturation3/1
  Saturation4/1 -> Mux2/5
  Torque/1 -> Saturation4/1
  Saturation2/1 -> Mux2/3
  Saturation3/1 -> Mux2/4
  Mux2/1 -> Out1/1

== system hip_controller_2026_01_07/Subsystem3/Left Motor Velocity/Subsystem/Subsystem2/Subsystem2 ==
  Kd1 : Constant  Value=5  OutDataTypeStr=single
  Kp1 : Constant  Value=500  OutDataTypeStr=single
  Position Command1 : Constant  Value=12.5  VectorParams1D=off  OutDataTypeStr=single
  Velocity Command1 : Constant  Value=45  OutDataTypeStr=single
  Out1 : Outport
  Out2 : Outport  Port=2
  Out3 : Outport  Port=3
  Out4 : Outport  Port=4
  wires:
  Kd1/1 -> Out4/1
  Position Command1/1 -> Out1/1
  Velocity Command1/1 -> Out2/1
  Kp1/1 -> Out3/1

== system hip_controller_2026_01_07/Subsystem3/Right Motor Velocity/Motor Actual Position Receive/CHINESE CORRECTION/Subsystem ==
  In1 : Inport
  Enable : EnablePort
  Memory : Memory
  Sum : Sum  Inputs=|++
  Out1 : Outport
  wires:
  In1/1 -> Sum/1
  Sum/1 -> Out1/1, Memory/1
  Memory/1 -> Sum/2

== system hip_controller_2026_01_07/Subsystem3/Right Motor Velocity/Motor Actual Position Receive/Unpack2/Subsystem ==
  In1 : Inport
  In2 : Inport  Port=2
  In3 : Inport  Port=3
  In4 : Inport  Port=4
  In5 : Inport  Port=5
  Bitwise AND : simulink/Logic and Bit Operations/Bitwise Operator  logicop=AND  UseBitMask=on  BitMask=bin2dec('0000000000001111')  BitMaskRealWorld=Stored Integer
  Bitwise OR : simulink/Logic and Bit Operations/Bitwise Operator  logicop=OR  UseBitMask=off  NumInputPorts=2  BitMask=bin2dec('11011001')  BitMaskRealWorld=Stored Integer
  Bitwise OR1 : simulink/Logic and Bit Operations/Bitwise Operator  logicop=OR  UseBitMask=off  NumInputPorts=2  BitMask=bin2dec('11011001')  BitMaskRealWorld=Stored Integer
  Bitwise OR2 : simulink/Logic and Bit Operations/Bitwise Operator  logicop=OR  UseBitMask=off  NumInputPorts=2  BitMask=bin2dec('11011001')  BitMaskRealWorld=Stored Integer
  Constant : Constant  Value=8  OutDataTypeStr=uint16
  Constant1 : Constant  Value=4  OutDataTypeStr=uint16
  Constant2 : Constant  Value=4  OutDataTypeStr=uint16
  Constant4 : Constant  Value=8  OutDataTypeStr=uint16
  Shift Arithmetic1 : ArithShift  BitShiftNumberSource=Input port  BitShiftNumber=8  BitShiftDirection=Left
      settings: InputPortMap=u0,p1
  Shift Arithmetic2 : ArithShift  BitShiftNumberSource=Input port  BitShiftNumber=8  BitShiftDirection=Left
      settings: InputPortMap=u0,p1
  Shift Arithmetic3 : ArithShift  BitShiftNumberSource=Input port  BitShiftNumber=8  BitShiftDirection=Right
      settings: InputPortMap=u0,p1
  Shift Arithmetic4 : ArithShift  BitShiftNumberSource=Input port  BitShiftNumber=8  BitShiftDirection=Left
      settings: InputPortMap=u0,p1
  Out1 : Outport
  Out2 : Outport  Port=2
  Out3 : Outport  Port=3
  wires:
  Bitwise AND/1 -> Shift Arithmetic4/1
  In5/1 -> Bitwise OR2/1
  Shift Arithmetic1/1 -> Bitwise OR1/1
  In1/1 -> Shift Arithmetic1/1
  Shift Arithmetic2/1 -> Bitwise OR/1
  Shift Arithmetic3/1 -> Bitwise OR/2
  Shift Arithmetic4/1 -> Bitwise OR2/2
  In2/1 -> Bitwise OR1/2
  Bitwise OR1/1 -> Out1/1
  Bitwise OR2/1 -> Out3/1
  In3/1 -> Shift Arithmetic2/1
  Constant4/1 -> Shift Arithmetic4/2
  Constant2/1 -> Shift Arithmetic3/2
  Constant1/1 -> Shift Arithmetic2/2
  Constant/1 -> Shift Arithmetic1/2
  Bitwise OR/1 -> Out2/1
  In4/1 -> Shift Arithmetic3/1, Bitwise AND/1

== system hip_controller_2026_01_07/Subsystem3/Right Motor Velocity/Subsystem/CAN Pack1/Subsystem ==
  p_int : Inport
  v_int : Inport  Port=2
  kp_int : Inport  Port=3
  kd_int : Inport  Port=4
  t_int : Inport  Port=5
  Buff 0 : Subsystem
  Buff 1 : Subsystem
  Buff 2 : Subsystem
  Buff 3 : Subsystem
  Buff 4 : Subsystem
  Buff 5 : Subsystem
  Buff 6 : Subsystem
  Buff 7 : Subsystem
  Out2 : Outport
  Out1 : Outport  Port=2
  Out3 : Outport  Port=3
  Out4 : Outport  Port=4
  Out5 : Outport  Port=5
  Out6 : Outport  Port=6
  Out7 : Outport  Port=7
  Out8 : Outport  Port=8
  wires:
  Buff 5/1(Out1) -> Out6/1
  Buff 7/1(Out1) -> Out8/1
  Buff 6/1(Out1) -> Out7/1
  Buff 0/1(Out1) -> Out2/1
  Buff 1/1(Out1) -> Out1/1
  Buff 2/1(Out1) -> Out3/1
  Buff 4/1(Out1) -> Out5/1
  Buff 3/1(Out1) -> Out4/1
  p_int/1 -> Buff 0/1(In1), Buff 1/1(In1)
  v_int/1 -> Buff 3/1(In1), Buff 2/1(In1)
  kd_int/1 -> Buff 6/1(In3), Buff 5/1(In2)
  kp_int/1 -> Buff 3/2(In2), Buff 4/1(In1)
  t_int/1 -> Buff 7/1(In1), Buff 6/2(In4)

== system hip_controller_2026_01_07/Subsystem3/Right Motor Velocity/Subsystem/Subsystem2/Subsystem ==
  In1 : Inport
  Kd : Constant  OutDataTypeStr=single
  Kp : Constant  Value=0  OutDataTypeStr=single
  Mux2 : Mux  Inputs=5
  Position Command : Constant  Value=0  VectorParams1D=off  OutDataTypeStr=single
  Saturation : Saturate  UpperLimit=12.5  LowerLimit=-12.5
  Saturation1 : Saturate  UpperLimit=41.87  LowerLimit=-41.87
  Saturation2 : Saturate  UpperLimit=500  LowerLimit=0
  Saturation3 : Saturate  UpperLimit=5  LowerLimit=0
  Saturation4 : Saturate  UpperLimit=9  LowerLimit=-9
  Torque : Constant  Value=0  OutDataTypeStr=single
  Out1 : Outport
  wires:
  Saturation/1 -> Mux2/1
  Kp/1 -> Saturation2/1
  In1/1 -> Saturation1/1
  Position Command/1 -> Saturation/1
  Saturation1/1 -> Mux2/2
  Kd/1 -> Saturation3/1
  Saturation4/1 -> Mux2/5
  Torque/1 -> Saturation4/1
  Saturation2/1 -> Mux2/3
  Saturation3/1 -> Mux2/4
  Mux2/1 -> Out1/1

== system hip_controller_2026_01_07/Subsystem3/Right Motor Velocity/Subsystem/Subsystem2/Subsystem2 ==
  Kd1 : Constant  Value=5  OutDataTypeStr=single
  Kp1 : Constant  Value=500  OutDataTypeStr=single
  Position Command1 : Constant  Value=12.5  VectorParams1D=off  OutDataTypeStr=single
  Velocity Command1 : Constant  Value=45  OutDataTypeStr=single
  Out1 : Outport
  Out2 : Outport  Port=2
  Out3 : Outport  Port=3
  Out4 : Outport  Port=4
  wires:
  Kd1/1 -> Out4/1
  Position Command1/1 -> Out1/1
  Velocity Command1/1 -> Out2/1
  Kp1/1 -> Out3/1

== system hip_controller_2026_01_07/Subsystem4/Left Motor Velocity/Motor Actual Position Receive/CHINESE CORRECTION/Subsystem ==
  In1 : Inport
  Enable : EnablePort
  Memory : Memory
  Sum : Sum  Inputs=|++
  Out1 : Outport
  wires:
  In1/1 -> Sum/1
  Sum/1 -> Out1/1, Memory/1
  Memory/1 -> Sum/2

== system hip_controller_2026_01_07/Subsystem4/Left Motor Velocity/Motor Actual Position Receive/Unpack2/Subsystem ==
  In1 : Inport
  In2 : Inport  Port=2
  In3 : Inport  Port=3
  In4 : Inport  Port=4
  In5 : Inport  Port=5
  Bitwise AND : simulink/Logic and Bit Operations/Bitwise Operator  logicop=AND  UseBitMask=on  BitMask=bin2dec('0000000000001111')  BitMaskRealWorld=Stored Integer
  Bitwise OR : simulink/Logic and Bit Operations/Bitwise Operator  logicop=OR  UseBitMask=off  NumInputPorts=2  BitMask=bin2dec('11011001')  BitMaskRealWorld=Stored Integer
  Bitwise OR1 : simulink/Logic and Bit Operations/Bitwise Operator  logicop=OR  UseBitMask=off  NumInputPorts=2  BitMask=bin2dec('11011001')  BitMaskRealWorld=Stored Integer
  Bitwise OR2 : simulink/Logic and Bit Operations/Bitwise Operator  logicop=OR  UseBitMask=off  NumInputPorts=2  BitMask=bin2dec('11011001')  BitMaskRealWorld=Stored Integer
  Constant : Constant  Value=8  OutDataTypeStr=uint16
  Constant1 : Constant  Value=4  OutDataTypeStr=uint16
  Constant2 : Constant  Value=4  OutDataTypeStr=uint16
  Constant4 : Constant  Value=8  OutDataTypeStr=uint16
  Shift Arithmetic1 : ArithShift  BitShiftNumberSource=Input port  BitShiftNumber=8  BitShiftDirection=Left
      settings: InputPortMap=u0,p1
  Shift Arithmetic2 : ArithShift  BitShiftNumberSource=Input port  BitShiftNumber=8  BitShiftDirection=Left
      settings: InputPortMap=u0,p1
  Shift Arithmetic3 : ArithShift  BitShiftNumberSource=Input port  BitShiftNumber=8  BitShiftDirection=Right
      settings: InputPortMap=u0,p1
  Shift Arithmetic4 : ArithShift  BitShiftNumberSource=Input port  BitShiftNumber=8  BitShiftDirection=Left
      settings: InputPortMap=u0,p1
  Out1 : Outport
  Out2 : Outport  Port=2
  Out3 : Outport  Port=3
  wires:
  Bitwise AND/1 -> Shift Arithmetic4/1
  In5/1 -> Bitwise OR2/1
  Shift Arithmetic1/1 -> Bitwise OR1/1
  In1/1 -> Shift Arithmetic1/1
  Shift Arithmetic2/1 -> Bitwise OR/1
  Shift Arithmetic3/1 -> Bitwise OR/2
  Shift Arithmetic4/1 -> Bitwise OR2/2
  In2/1 -> Bitwise OR1/2
  Bitwise OR1/1 -> Out1/1
  Bitwise OR2/1 -> Out3/1
  In3/1 -> Shift Arithmetic2/1
  Constant4/1 -> Shift Arithmetic4/2
  Constant2/1 -> Shift Arithmetic3/2
  Constant1/1 -> Shift Arithmetic2/2
  Constant/1 -> Shift Arithmetic1/2
  Bitwise OR/1 -> Out2/1
  In4/1 -> Shift Arithmetic3/1, Bitwise AND/1

== system hip_controller_2026_01_07/Subsystem4/Left Motor Velocity/Subsystem/CAN Pack1/Subsystem ==
  p_int : Inport
  v_int : Inport  Port=2
  kp_int : Inport  Port=3
  kd_int : Inport  Port=4
  t_int : Inport  Port=5
  Buff 0 : Subsystem
  Buff 1 : Subsystem
  Buff 2 : Subsystem
  Buff 3 : Subsystem
  Buff 4 : Subsystem
  Buff 5 : Subsystem
  Buff 6 : Subsystem
  Buff 7 : Subsystem
  Out2 : Outport
  Out1 : Outport  Port=2
  Out3 : Outport  Port=3
  Out4 : Outport  Port=4
  Out5 : Outport  Port=5
  Out6 : Outport  Port=6
  Out7 : Outport  Port=7
  Out8 : Outport  Port=8
  wires:
  Buff 5/1(Out1) -> Out6/1
  Buff 7/1(Out1) -> Out8/1
  Buff 6/1(Out1) -> Out7/1
  Buff 0/1(Out1) -> Out2/1
  Buff 1/1(Out1) -> Out1/1
  Buff 2/1(Out1) -> Out3/1
  Buff 4/1(Out1) -> Out5/1
  Buff 3/1(Out1) -> Out4/1
  p_int/1 -> Buff 0/1(In1), Buff 1/1(In1)
  v_int/1 -> Buff 3/1(In1), Buff 2/1(In1)
  kd_int/1 -> Buff 6/1(In3), Buff 5/1(In2)
  kp_int/1 -> Buff 3/2(In2), Buff 4/1(In1)
  t_int/1 -> Buff 7/1(In1), Buff 6/2(In4)

== system hip_controller_2026_01_07/Subsystem4/Left Motor Velocity/Subsystem/Subsystem2/Subsystem ==
  In1 : Inport
  Kd : Constant  OutDataTypeStr=single
  Kp : Constant  Value=0  OutDataTypeStr=single
  Mux2 : Mux  Inputs=5
  Position Command : Constant  Value=0  VectorParams1D=off  OutDataTypeStr=single
  Saturation : Saturate  UpperLimit=12.5  LowerLimit=-12.5
  Saturation1 : Saturate  UpperLimit=41.87  LowerLimit=-41.87
  Saturation2 : Saturate  UpperLimit=500  LowerLimit=0
  Saturation3 : Saturate  UpperLimit=5  LowerLimit=0
  Saturation4 : Saturate  UpperLimit=9  LowerLimit=-9
  Torque : Constant  Value=0  OutDataTypeStr=single
  Out1 : Outport
  wires:
  Saturation/1 -> Mux2/1
  Kp/1 -> Saturation2/1
  In1/1 -> Saturation1/1
  Position Command/1 -> Saturation/1
  Saturation1/1 -> Mux2/2
  Kd/1 -> Saturation3/1
  Saturation4/1 -> Mux2/5
  Torque/1 -> Saturation4/1
  Saturation2/1 -> Mux2/3
  Saturation3/1 -> Mux2/4
  Mux2/1 -> Out1/1

== system hip_controller_2026_01_07/Subsystem4/Left Motor Velocity/Subsystem/Subsystem2/Subsystem2 ==
  Kd1 : Constant  Value=5  OutDataTypeStr=single
  Kp1 : Constant  Value=500  OutDataTypeStr=single
  Position Command1 : Constant  Value=12.5  VectorParams1D=off  OutDataTypeStr=single
  Velocity Command1 : Constant  Value=45  OutDataTypeStr=single
  Out1 : Outport
  Out2 : Outport  Port=2
  Out3 : Outport  Port=3
  Out4 : Outport  Port=4
  wires:
  Kd1/1 -> Out4/1
  Position Command1/1 -> Out1/1
  Velocity Command1/1 -> Out2/1
  Kp1/1 -> Out3/1

== system hip_controller_2026_01_07/Subsystem4/Right Motor Velocity/Motor Actual Position Receive/CHINESE CORRECTION/Subsystem ==
  In1 : Inport
  Enable : EnablePort
  Memory : Memory
  Sum : Sum  Inputs=|++
  Out1 : Outport
  wires:
  In1/1 -> Sum/1
  Sum/1 -> Out1/1, Memory/1
  Memory/1 -> Sum/2

== system hip_controller_2026_01_07/Subsystem4/Right Motor Velocity/Motor Actual Position Receive/Unpack2/Subsystem ==
  In1 : Inport
  In2 : Inport  Port=2
  In3 : Inport  Port=3
  In4 : Inport  Port=4
  In5 : Inport  Port=5
  Bitwise AND : simulink/Logic and Bit Operations/Bitwise Operator  logicop=AND  UseBitMask=on  BitMask=bin2dec('0000000000001111')  BitMaskRealWorld=Stored Integer
  Bitwise OR : simulink/Logic and Bit Operations/Bitwise Operator  logicop=OR  UseBitMask=off  NumInputPorts=2  BitMask=bin2dec('11011001')  BitMaskRealWorld=Stored Integer
  Bitwise OR1 : simulink/Logic and Bit Operations/Bitwise Operator  logicop=OR  UseBitMask=off  NumInputPorts=2  BitMask=bin2dec('11011001')  BitMaskRealWorld=Stored Integer
  Bitwise OR2 : simulink/Logic and Bit Operations/Bitwise Operator  logicop=OR  UseBitMask=off  NumInputPorts=2  BitMask=bin2dec('11011001')  BitMaskRealWorld=Stored Integer
  Constant : Constant  Value=8  OutDataTypeStr=uint16
  Constant1 : Constant  Value=4  OutDataTypeStr=uint16
  Constant2 : Constant  Value=4  OutDataTypeStr=uint16
  Constant4 : Constant  Value=8  OutDataTypeStr=uint16
  Shift Arithmetic1 : ArithShift  BitShiftNumberSource=Input port  BitShiftNumber=8  BitShiftDirection=Left
      settings: InputPortMap=u0,p1
  Shift Arithmetic2 : ArithShift  BitShiftNumberSource=Input port  BitShiftNumber=8  BitShiftDirection=Left
      settings: InputPortMap=u0,p1
  Shift Arithmetic3 : ArithShift  BitShiftNumberSource=Input port  BitShiftNumber=8  BitShiftDirection=Right
      settings: InputPortMap=u0,p1
  Shift Arithmetic4 : ArithShift  BitShiftNumberSource=Input port  BitShiftNumber=8  BitShiftDirection=Left
      settings: InputPortMap=u0,p1
  Out1 : Outport
  Out2 : Outport  Port=2
  Out3 : Outport  Port=3
  wires:
  Bitwise AND/1 -> Shift Arithmetic4/1
  In5/1 -> Bitwise OR2/1
  Shift Arithmetic1/1 -> Bitwise OR1/1
  In1/1 -> Shift Arithmetic1/1
  Shift Arithmetic2/1 -> Bitwise OR/1
  Shift Arithmetic3/1 -> Bitwise OR/2
  Shift Arithmetic4/1 -> Bitwise OR2/2
  In2/1 -> Bitwise OR1/2
  Bitwise OR1/1 -> Out1/1
  Bitwise OR2/1 -> Out3/1
  In3/1 -> Shift Arithmetic2/1
  Constant4/1 -> Shift Arithmetic4/2
  Constant2/1 -> Shift Arithmetic3/2
  Constant1/1 -> Shift Arithmetic2/2
  Constant/1 -> Shift Arithmetic1/2
  Bitwise OR/1 -> Out2/1
  In4/1 -> Shift Arithmetic3/1, Bitwise AND/1

== system hip_controller_2026_01_07/Subsystem4/Right Motor Velocity/Subsystem/CAN Pack1/Subsystem ==
  p_int : Inport
  v_int : Inport  Port=2
  kp_int : Inport  Port=3
  kd_int : Inport  Port=4
  t_int : Inport  Port=5
  Buff 0 : Subsystem
  Buff 1 : Subsystem
  Buff 2 : Subsystem
  Buff 3 : Subsystem
  Buff 4 : Subsystem
  Buff 5 : Subsystem
  Buff 6 : Subsystem
  Buff 7 : Subsystem
  Out2 : Outport
  Out1 : Outport  Port=2
  Out3 : Outport  Port=3
  Out4 : Outport  Port=4
  Out5 : Outport  Port=5
  Out6 : Outport  Port=6
  Out7 : Outport  Port=7
  Out8 : Outport  Port=8
  wires:
  Buff 5/1(Out1) -> Out6/1
  Buff 7/1(Out1) -> Out8/1
  Buff 6/1(Out1) -> Out7/1
  Buff 0/1(Out1) -> Out2/1
  Buff 1/1(Out1) -> Out1/1
  Buff 2/1(Out1) -> Out3/1
  Buff 4/1(Out1) -> Out5/1
  Buff 3/1(Out1) -> Out4/1
  p_int/1 -> Buff 0/1(In1), Buff 1/1(In1)
  v_int/1 -> Buff 3/1(In1), Buff 2/1(In1)
  kd_int/1 -> Buff 6/1(In3), Buff 5/1(In2)
  kp_int/1 -> Buff 3/2(In2), Buff 4/1(In1)
  t_int/1 -> Buff 7/1(In1), Buff 6/2(In4)

== system hip_controller_2026_01_07/Subsystem4/Right Motor Velocity/Subsystem/Subsystem2/Subsystem ==
  In1 : Inport
  Kd : Constant  OutDataTypeStr=single
  Kp : Constant  Value=0  OutDataTypeStr=single
  Mux2 : Mux  Inputs=5
  Position Command : Constant  Value=0  VectorParams1D=off  OutDataTypeStr=single
  Saturation : Saturate  UpperLimit=12.5  LowerLimit=-12.5
  Saturation1 : Saturate  UpperLimit=41.87  LowerLimit=-41.87
  Saturation2 : Saturate  UpperLimit=500  LowerLimit=0
  Saturation3 : Saturate  UpperLimit=5  LowerLimit=0
  Saturation4 : Saturate  UpperLimit=9  LowerLimit=-9
  Torque : Constant  Value=0  OutDataTypeStr=single
  Out1 : Outport
  wires:
  Saturation/1 -> Mux2/1
  Kp/1 -> Saturation2/1
  In1/1 -> Saturation1/1
  Position Command/1 -> Saturation/1
  Saturation1/1 -> Mux2/2
  Kd/1 -> Saturation3/1
  Saturation4/1 -> Mux2/5
  Torque/1 -> Saturation4/1
  Saturation2/1 -> Mux2/3
  Saturation3/1 -> Mux2/4
  Mux2/1 -> Out1/1

== system hip_controller_2026_01_07/Subsystem4/Right Motor Velocity/Subsystem/Subsystem2/Subsystem2 ==
  Kd1 : Constant  Value=5  OutDataTypeStr=single
  Kp1 : Constant  Value=500  OutDataTypeStr=single
  Position Command1 : Constant  Value=12.5  VectorParams1D=off  OutDataTypeStr=single
  Velocity Command1 : Constant  Value=45  OutDataTypeStr=single
  Out1 : Outport
  Out2 : Outport  Port=2
  Out3 : Outport  Port=3
  Out4 : Outport  Port=4
  wires:
  Kd1/1 -> Out4/1
  Position Command1/1 -> Out1/1
  Velocity Command1/1 -> Out2/1
  Kp1/1 -> Out3/1

== system hip_controller_2026_01_07/Subsystem3/Left Motor Velocity/Subsystem/CAN Pack1/Subsystem/Buff 0 ==
  In1 : Inport
  Constant1 : Constant  Value=8  OutDataTypeStr=uint16
  Data Type Conversion : DataTypeConversion  OutDataTypeStr=uint8  SaturateOnIntegerOverflow=off  RndMeth=Floor
  Shift Arithmetic2 : ArithShift  BitShiftNumberSource=Input port  BitShiftNumber=8  BitShiftDirection=Right
      settings: InputPortMap=u0,p1
  Out1 : Outport
  wires:
  In1/1 -> Shift Arithmetic2/1
  Shift Arithmetic2/1 -> Data Type Conversion/1
  Data Type Conversion/1 -> Out1/1
  Constant1/1 -> Shift Arithmetic2/2

== system hip_controller_2026_01_07/Subsystem3/Left Motor Velocity/Subsystem/CAN Pack1/Subsystem/Buff 1 ==
  In1 : Inport
  Bitwise AND : simulink/Logic and Bit Operations/Bitwise Operator  logicop=AND  UseBitMask=on  BitMask=bin2dec('0000000011111111')  BitMaskRealWorld=Stored Integer
  Data Type Conversion1 : DataTypeConversion  OutDataTypeStr=uint8  SaturateOnIntegerOverflow=off  RndMeth=Floor
  Out1 : Outport
  wires:
  Bitwise AND/1 -> Data Type Conversion1/1
  Data Type Conversion1/1 -> Out1/1
  In1/1 -> Bitwise AND/1

== system hip_controller_2026_01_07/Subsystem3/Left Motor Velocity/Subsystem/CAN Pack1/Subsystem/Buff 2 ==
  In1 : Inport
  Constant2 : Constant  Value=4  OutDataTypeStr=uint16
  Data Type Conversion2 : DataTypeConversion  OutDataTypeStr=uint8  SaturateOnIntegerOverflow=off  RndMeth=Floor
  Shift Arithmetic1 : ArithShift  BitShiftNumberSource=Input port  BitShiftNumber=8  BitShiftDirection=Right
      settings: InputPortMap=u0,p1
  Out1 : Outport
  wires:
  Shift Arithmetic1/1 -> Data Type Conversion2/1
  Data Type Conversion2/1 -> Out1/1
  In1/1 -> Shift Arithmetic1/1
  Constant2/1 -> Shift Arithmetic1/2

== system hip_controller_2026_01_07/Subsystem3/Left Motor Velocity/Subsystem/CAN Pack1/Subsystem/Buff 3 ==
  In1 : Inport
  In2 : Inport  Port=2
  Bitwise AND1 : simulink/Logic and Bit Operations/Bitwise Operator  logicop=AND  UseBitMask=on  BitMask=bin2dec('000000001111')  BitMaskRealWorld=Stored Integer
  Bitwise OR1 : simulink/Logic and Bit Operations/Bitwise Operator  logicop=OR  UseBitMask=off  NumInputPorts=2  BitMask=bin2dec('11011001')  BitMaskRealWorld=Stored Integer
  Constant1 : Constant  Value=8  OutDataTypeStr=uint16
  Constant2 : Constant  Value=4  OutDataTypeStr=uint16
  Data Type Conversion3 : DataTypeConversion  OutDataTypeStr=uint8  SaturateOnIntegerOverflow=off  RndMeth=Floor
  Shift Arithmetic3 : ArithShift  BitShiftNumberSource=Input port  BitShiftNumber=8  BitShiftDirection=Left
      settings: InputPortMap=u0,p1
  Shift Arithmetic4 : ArithShift  BitShiftNumberSource=Input port  BitShiftNumber=8  BitShiftDirection=Right
      settings: InputPortMap=u0,p1
  Out1 : Outport
  wires:
  Shift Arithmetic3/1 -> Bitwise OR1/1
  In1/1 -> Bitwise AND1/1
  Constant1/1 -> Shift Arithmetic4/2
  Bitwise AND1/1 -> Shift Arithmetic3/1
  Shift Arithmetic4/1 -> Bitwise OR1/2
  In2/1 -> Shift Arithmetic4/1
  Bitwise OR1/1 -> Data Type Conversion3/1
  Data Type Conversion3/1 -> Out1/1
  Constant2/1 -> Shift Arithmetic3/2

== system hip_controller_2026_01_07/Subsystem3/Left Motor Velocity/Subsystem/CAN Pack1/Subsystem/Buff 4 ==
  In1 : Inport
  Bitwise AND3 : simulink/Logic and Bit Operations/Bitwise Operator  logicop=AND  UseBitMask=on  BitMask=bin2dec('000011111111')  BitMaskRealWorld=Stored Integer
  Data Type Conversion4 : DataTypeConversion  OutDataTypeStr=uint8  SaturateOnIntegerOverflow=off  RndMeth=Floor
  Out1 : Outport
  wires:
  Data Type Conversion4/1 -> Out1/1
  Bitwise AND3/1 -> Data Type Conversion4/1
  In1/1 -> Bitwise AND3/1

== system hip_controller_2026_01_07/Subsystem3/Left Motor Velocity/Subsystem/CAN Pack1/Subsystem/Buff 5 ==
  In2 : Inport
  Constant2 : Constant  Value=4  OutDataTypeStr=uint16
  Data Type Conversion5 : DataTypeConversion  OutDataTypeStr=uint8  SaturateOnIntegerOverflow=off  RndMeth=Floor
  Shift Arithmetic5 : ArithShift  BitShiftNumberSource=Input port  BitShiftNumber=8  BitShiftDirection=Right
      settings: InputPortMap=u0,p1
  Out1 : Outport
  wires:
  In2/1 -> Shift Arithmetic5/1
  Shift Arithmetic5/1 -> Data Type Conversion5/1
  Data Type Conversion5/1 -> Out1/1
  Constant2/1 -> Shift Arithmetic5/2

== system hip_controller_2026_01_07/Subsystem3/Left Motor Velocity/Subsystem/CAN Pack1/Subsystem/Buff 6 ==
  In3 : Inport
  In4 : Inport  Port=2
  Bitwise AND2 : simulink/Logic and Bit Operations/Bitwise Operator  logicop=AND  UseBitMask=on  BitMask=bin2dec('000000001111')  BitMaskRealWorld=Stored Integer
  Bitwise OR2 : simulink/Logic and Bit Operations/Bitwise Operator  logicop=OR  UseBitMask=off  NumInputPorts=2  BitMask=bin2dec('11011001')  BitMaskRealWorld=Stored Integer
  Constant1 : Constant  Value=8  OutDataTypeStr=uint16
  Constant2 : Constant  Value=4  OutDataTypeStr=uint16
  Data Type Conversion6 : DataTypeConversion  OutDataTypeStr=uint8  SaturateOnIntegerOverflow=off  RndMeth=Floor
  Shift Arithmetic6 : ArithShift  BitShiftNumberSource=Input port  BitShiftNumber=8  BitShiftDirection=Left
      settings: InputPortMap=u0,p1
  Shift Arithmetic7 : ArithShift  BitShiftNumberSource=Input port  BitShiftNumber=8  BitShiftDirection=Right
      settings: InputPortMap=u0,p1
  Out1 : Outport
  wires:
  In4/1 -> Shift Arithmetic7/1
  Shift Arithmetic7/1 -> Bitwise OR2/2
  Shift Arithmetic6/1 -> Bitwise OR2/1
  Bitwise OR2/1 -> Data Type Conversion6/1
  In3/1 -> Bitwise AND2/1
  Bitwise AND2/1 -> Shift Arithmetic6/1
  Data Type Conversion6/1 -> Out1/1
  Constant2/1 -> Shift Arithmetic6/2
  Constant1/1 -> Shift Arithmetic7/2

== system hip_controller_2026_01_07/Subsystem3/Left Motor Velocity/Subsystem/CAN Pack1/Subsystem/Buff 7 ==
  In1 : Inport
  Bitwise AND4 : simulink/Logic and Bit Operations/Bitwise Operator  logicop=AND  UseBitMask=on  BitMask=bin2dec('000011111111')  BitMaskRealWorld=Stored Integer
  Data Type Conversion7 : DataTypeConversion  OutDataTypeStr=uint8  SaturateOnIntegerOverflow=off  RndMeth=Floor
  Out1 : Outport
  wires:
  Bitwise AND4/1 -> Data Type Conversion7/1
  Data Type Conversion7/1 -> Out1/1
  In1/1 -> Bitwise AND4/1

== system hip_controller_2026_01_07/Subsystem3/Right Motor Velocity/Subsystem/CAN Pack1/Subsystem/Buff 0 ==
  In1 : Inport
  Constant1 : Constant  Value=8  OutDataTypeStr=uint16
  Data Type Conversion : DataTypeConversion  OutDataTypeStr=uint8  SaturateOnIntegerOverflow=off  RndMeth=Floor
  Shift Arithmetic2 : ArithShift  BitShiftNumberSource=Input port  BitShiftNumber=8  BitShiftDirection=Right
      settings: InputPortMap=u0,p1
  Out1 : Outport
  wires:
  In1/1 -> Shift Arithmetic2/1
  Shift Arithmetic2/1 -> Data Type Conversion/1
  Data Type Conversion/1 -> Out1/1
  Constant1/1 -> Shift Arithmetic2/2

== system hip_controller_2026_01_07/Subsystem3/Right Motor Velocity/Subsystem/CAN Pack1/Subsystem/Buff 1 ==
  In1 : Inport
  Bitwise AND : simulink/Logic and Bit Operations/Bitwise Operator  logicop=AND  UseBitMask=on  BitMask=bin2dec('0000000011111111')  BitMaskRealWorld=Stored Integer
  Data Type Conversion1 : DataTypeConversion  OutDataTypeStr=uint8  SaturateOnIntegerOverflow=off  RndMeth=Floor
  Out1 : Outport
  wires:
  Bitwise AND/1 -> Data Type Conversion1/1
  Data Type Conversion1/1 -> Out1/1
  In1/1 -> Bitwise AND/1
